simulink model "PID_Controller_Design"  (R2020a)
settings: Solver=VariableStepAuto  StartTime=0.0  StopTime=10.0  RelTol=1e-3
values from neighbouring files (symbols this model uses):
  wn = 1/RC    (= 1250)    [secend_order_closed_loop.m]
  zeta = 1    [secend_order_closed_loop.m]
settings Model: Creator=Administrator  LastModifiedBy=Administrator

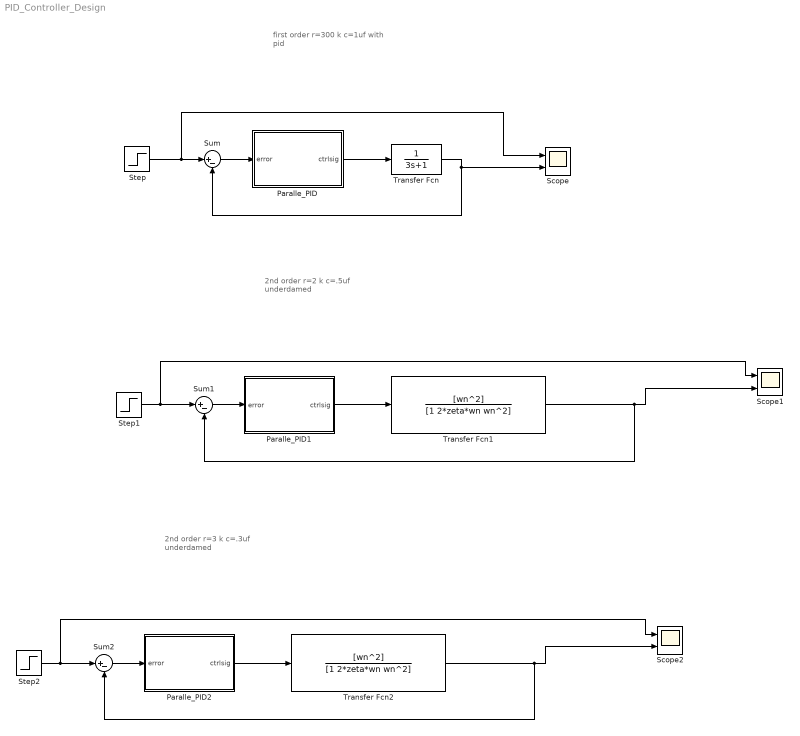
== system PID_Controller_Design ==
  note: first order
      | r=300 k
      | c=1uf
      | with pid
  note: 2nd order
      | r=2 k
      | c=.5uf
      | underdamed
  note: 2nd order
      | r=3 k
      | c=.3uf
      | underdamed
  Paralle_PID : Subsystem
  Paralle_PID1 : Subsystem
  Paralle_PID2 : Subsystem
  Scope : Scope  NumInputPorts=2
  Scope1 : Scope  NumInputPorts=2
  Scope2 : Scope  NumInputPorts=2
  Step : Step  SampleTime=0
  Step1 : Step  SampleTime=0
  Step2 : Step  SampleTime=0
  Sum : Sum  Inputs=|+-
  Sum1 : Sum  Inputs=|+-
  Sum2 : Sum  Inputs=|+-
  Transfer Fcn : TransferFcn  Denominator=[3 1]
  Transfer Fcn1 : TransferFcn  Numerator=[wn^2]  Denominator=[1 2*zeta*wn wn^2]
  Transfer Fcn2 : TransferFcn  Numerator=[wn^2]  Denominator=[1 2*zeta*wn wn^2]
  wires:
  Paralle_PID/1(ctrlsig) -> Transfer Fcn/1
  Transfer Fcn/1 -> Scope/2, Sum/2
  Step/1 -> Scope/1, Sum/1
  Sum/1 -> Paralle_PID/1(error)
  Sum1/1 -> Paralle_PID1/1(error)
  Step1/1 -> Scope1/1, Sum1/1
  Paralle_PID1/1(ctrlsig) -> Transfer Fcn1/1
  Transfer Fcn1/1 -> Sum1/2, Scope1/2
  Transfer Fcn2/1 -> Scope2/2, Sum2/2
  Paralle_PID2/1(ctrlsig) -> Transfer Fcn2/1
  Step2/1 -> Sum2/1, Scope2/1
  Sum2/1 -> Paralle_PID2/1(error)

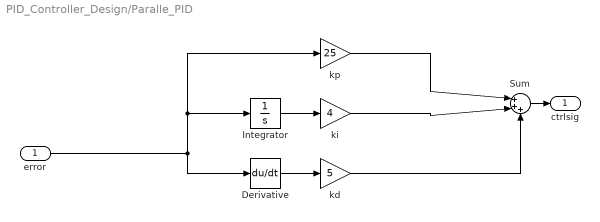
== system PID_Controller_Design/Paralle_PID ==
  error : Inport
  Derivative : Derivative
  Integrator : Integrator
  Sum : Sum  Inputs=|+++
  kd : Gain  Gain=5
  ki : Gain  Gain=4
  kp : Gain  Gain=25
  ctrlsig : Outport
  wires:
  error/1 -> Derivative/1, Integrator/1, kp/1
  ki/1 -> Sum/2
  Integrator/1 -> ki/1
  Sum/1 -> ctrlsig/1
  Derivative/1 -> kd/1
  kd/1 -> Sum/3
  kp/1 -> Sum/1

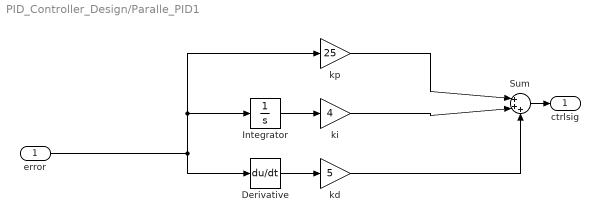
== system PID_Controller_Design/Paralle_PID1 ==
  error : Inport
  Derivative : Derivative
  Integrator : Integrator
  Sum : Sum  Inputs=|+++
  kd : Gain  Gain=5
  ki : Gain  Gain=4
  kp : Gain  Gain=25
  ctrlsig : Outport
  wires:
  kp/1 -> Sum/1
  kd/1 -> Sum/3
  Derivative/1 -> kd/1
  Sum/1 -> ctrlsig/1
  Integrator/1 -> ki/1
  ki/1 -> Sum/2
  error/1 -> kp/1, Integrator/1, Derivative/1

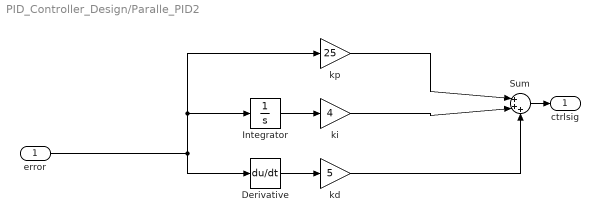
== system PID_Controller_Design/Paralle_PID2 ==
  error : Inport
  Derivative : Derivative
  Integrator : Integrator
  Sum : Sum  Inputs=|+++
  kd : Gain  Gain=5
  ki : Gain  Gain=4
  kp : Gain  Gain=25
  ctrlsig : Outport
  wires:
  error/1 -> Derivative/1, Integrator/1, kp/1
  ki/1 -> Sum/2
  Integrator/1 -> ki/1
  Sum/1 -> ctrlsig/1
  Derivative/1 -> kd/1
  kd/1 -> Sum/3
  kp/1 -> Sum/1
